simulink model "Timers"  (R2025a)
settings: Solver=FixedStepDiscrete  StartTime=0  StopTime=1  FixedStep=1e-7  RelTol=1e-3
libraries: simulink_extras x216, simulink x13
(part 1 of 7)
settings Model: PacingRate=0.000500  Creator=Erys  LastModifiedBy=Erys
settings DebuggingCC: AlgebraicLoopMsg=none  ForceCombineOutputUpdateInSim=on

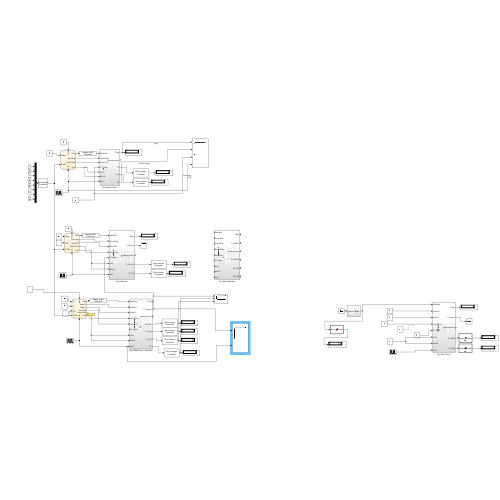
[thumbnail: Simulink's stored preview of the top-level diagram]
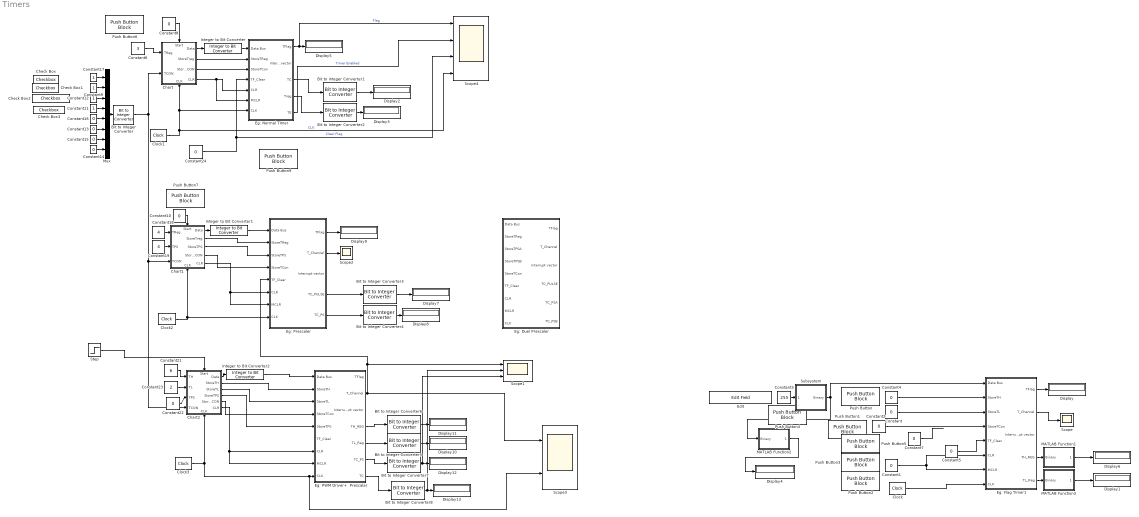
== system Timers ==
  Bit to Integer Converter : simulink/Logic and Bit Operations/Bit to Integer Converter  nbits=8  bitOrder=MSB first  signedOutputValues=Unsigned  outDtype=double  outDtypeSigned=Inherit via internal rule
  Bit to Integer Converter{1..8} (8 alike) : simulink/Logic and Bit Operations/Bit to Integer Converter  nbits=8  bitOrder=MSB first  signedOutputValues=Unsigned  outDtype=Inherit via internal rule  outDtypeSigned=Inherit via internal rule
  Chart : Stateflow chart  TreatAsAtomicUnit=on
      settings: PortSchema="{\"entries\":[{\"content\":{\"sides\":[{\"content\":{\"connectorIds\":[\"In4\",\"In1\"]},\"type\":\"ConnectorPlacement.EquallySpacedRectSide\",\"uuid\":\"e074c012-5276-4155-8d53-51c993f7710d\"},{\"content\":{\"connectorIds\":[\"Out2\",\"Out3\",\"Out4\",\"Out1\"],\"side\":\"RIGHT\"},\"type\":\"ConnectorPlacement.EquallySpacedRectSide\",\"uuid\":\"84a6596f-ad90-40d7-98bc-5213cd18cdfd\"},{\"content\":{\"connectorIds\":[\"In2\"],\"side\":\"TOP\"},\"type\":\"ConnectorPlacement.EquallySpacedRectSide\",\"uuid\":\"9e281591-ea24-4a8d-8cd5-85def40d3d51\"},{\"content\":{\"connectorIds\":[\"In3\"],\"side\":\"BOTTOM\"},\"type\":\"ConnectorPlacement.EquallySpacedRectSide\",\"uuid\":\"88479451-5760-4ccc-a9c9-4ac76de2b8f0\"}]},\"type\":\"ConnectorPlacement.EquallySpacedConnector\",\"uuid\":\"45dca767-207d-4cb9-a557-26c3450393e5\"}],\"packageUris\":[\"http://schema.mathworks.com/mf0/Connector/R2020b\"],\"version\":\"1.0\"}"
  Chart1 : Stateflow chart  TreatAsAtomicUnit=on
      settings: PortSchema="{\"entries\":[{\"content\":{\"sides\":[{\"content\":{\"connectorIds\":[\"In4\",\"In5\",\"In1\"]},\"type\":\"ConnectorPlacement.EquallySpacedRectSide\",\"uuid\":\"e074c012-5276-4155-8d53-51c993f7710d\"},{\"content\":{\"connectorIds\":[\"Out2\",\"Out4\",\"Out3\",\"Out5\",\"Out1\"],\"side\":\"RIGHT\"},\"type\":\"ConnectorPlacement.EquallySpacedRectSide\",\"uuid\":\"84a6596f-ad90-40d7-98bc-5213cd18cdfd\"},{\"content\":{\"connectorIds\":[\"In2\"],\"side\":\"TOP\"},\"type\":\"ConnectorPlacement.EquallySpacedRectSide\",\"uuid\":\"9e281591-ea24-4a8d-8cd5-85def40d3d51\"},{\"content\":{\"connectorIds\":[\"In3\"],\"side\":\"BOTTOM\"},\"type\":\"ConnectorPlacement.EquallySpacedRectSide\",\"uuid\":\"88479451-5760-4ccc-a9c9-4ac76de2b8f0\"}]},\"type\":\"ConnectorPlacement.EquallySpacedConnector\",\"uuid\":\"45dca767-207d-4cb9-a557-26c3450393e5\"}],\"packageUris\":[\"http://schema.mathworks.com/mf0/Connector/R2020b\"],\"version\":\"1.0\"}"
  Chart2 : Stateflow chart  TreatAsAtomicUnit=on
      settings: PortSchema="{\"entries\":[{\"content\":{\"sides\":[{\"content\":{\"connectorIds\":[\"In4\",\"In6\",\"In5\",\"In1\"]},\"type\":\"ConnectorPlacement.EquallySpacedRectSide\",\"uuid\":\"e074c012-5276-4155-8d53-51c993f7710d\"},{\"content\":{\"connectorIds\":[\"Out2\",\"Out5\",\"Out6\",\"Out3\",\"Out4\",\"Out1\"],\"side\":\"RIGHT\"},\"type\":\"ConnectorPlacement.EquallySpacedRectSide\",\"uuid\":\"84a6596f-ad90-40d7-98bc-5213cd18cdfd\"},{\"content\":{\"connectorIds\":[\"In2\"],\"side\":\"TOP\"},\"type\":\"ConnectorPlacement.EquallySpacedRectSide\",\"uuid\":\"9e281591-ea24-4a8d-8cd5-85def40d3d51\"},{\"content\":{\"connectorIds\":[\"In3\"],\"side\":\"BOTTOM\"},\"type\":\"ConnectorPlacement.EquallySpacedRectSide\",\"uuid\":\"88479451-5760-4ccc-a9c9-4ac76de2b8f0\"}]},\"type\":\"ConnectorPlacement.EquallySpacedConnector\",\"uuid\":\"45dca767-207d-4cb9-a557-26c3450393e5\"}],\"packageUris\":[\"http://schema.mathworks.com/mf0/Connector/R2020b\"],\"version\":\"1.0\"}"
  Check Box : Checkbox  LabelPosition=Hide  ShowInitialText=on  Label=Enable  Values=[0.0, 1.0]
  Check Box1 : Checkbox  LabelPosition=Hide  ShowInitialText=on  Label=AutoReload  Values=[0.0, 1.0]
  Check Box2 : Checkbox  LabelPosition=Hide  ShowInitialText=on  Label=INterrupt  Values=[0.0, 1.0]
  Check Box3 : Checkbox  LabelPosition=Hide  ShowInitialText=on  Label=Gate  Values=[0.0, 1.0]
  Clock : simulink_extras/Flip Flops/Clock  period=0.01
  Clock1 : simulink_extras/Flip Flops/Clock  period=0.001
  Clock2 : simulink_extras/Flip Flops/Clock  period=0.0001
  Clock3 : simulink_extras/Flip Flops/Clock  period=0.0001
  Constant{,1..2,4..5,7,13..16} (10 alike) : Constant  Value=0  OutDataTypeStr=boolean
  Constant{8,10,22,24} (4 alike) : Constant  Value=0
  Constant{9,11..12,17} (4 alike) : Constant  OutDataTypeStr=boolean
  Constant18 : Constant  Value=4
  Constant19 : Constant  Value=4
  Constant21 : Constant  Value=6
  Constant23 : Constant  Value=2
  Constant3 : Constant  Value=255
  Constant6 : Constant  Value=3
  Display{,1..13} (14 alike) : Display
  Edit : EditField  LabelPosition=Hide  ShowInitialText=on  Alignment=Center
  Eg: Duel Prescaler : Subsystem
  Eg: Flag Timer1 : Subsystem
  Eg: Normal TImer : Subsystem
  Eg: PWM Driver+  Prescalar : Subsystem
  Eg: Prescaler : Subsystem
  Integer to Bit Converter : simulink/Logic and Bit Operations/Integer to Bit Converter  nbits=8  signedInputValues=Unsigned  bitOrder=MSB first  outDtype=Inherit via internal rule
  Integer to Bit Converter1 : simulink/Logic and Bit Operations/Integer to Bit Converter  nbits=8  signedInputValues=Unsigned  bitOrder=MSB first  outDtype=Inherit via internal rule
  Integer to Bit Converter2 : simulink/Logic and Bit Operations/Integer to Bit Converter  nbits=8  signedInputValues=Unsigned  bitOrder=MSB first  outDtype=Inherit via internal rule
  MATLAB Function1 : MATLAB Function  TreatAsAtomicUnit=on
  MATLAB Function2 : MATLAB Function  TreatAsAtomicUnit=on
  MATLAB Function3 : MATLAB Function  TreatAsAtomicUnit=on
  Mux : Mux  Inputs=8
  Push Button : PushButtonBlock  ButtonText=TH  IconOnColor=[0.0, 0.39215686274509803, 0.0]  IconOffColor=[0.0, 1.0, 0.0]  OffValue=0.000000
  Push Button1 : PushButtonBlock  ButtonText=T_CON  IconOnColor=[0.0, 0.39215686274509803, 0.0]  IconOffColor=[0.0, 1.0, 0.0]  OffValue=0.000000
  Push Button2 : PushButtonBlock  ButtonText=CLR  IconOnColor=[0.0, 0.39215686274509803, 0.0]  IconOffColor=[0.0, 1.0, 0.0]  OffValue=0.000000
  Push Button3 : PushButtonBlock  ButtonText=RST  IconOnColor=[0.0, 0.39215686274509803, 0.0]  IconOffColor=[0.0, 1.0, 0.0]  OffValue=0.000000
  Push Button4 : PushButtonBlock  ButtonText=TL  IconOnColor=[0.0, 0.39215686274509803, 0.0]  IconOffColor=[0.0, 1.0, 0.0]  OffValue=0.000000
  Push Button5 : PushButtonBlock  ButtonText=T_PSB  IconOnColor=[0.0, 0.39215686274509803, 0.0]  IconOffColor=[0.0, 1.0, 0.0]  OffValue=0.000000
  Push Button6 : PushButtonBlock  ButtonText=Start  IconOnColor=[0.0, 0.39215686274509803, 0.0]  IconOffColor=[0.0, 1.0, 0.0]  OffValue=0.000000
  Push Button7 : PushButtonBlock  ButtonText=Start  IconOnColor=[0.0, 0.39215686274509803, 0.0]  IconOffColor=[0.0, 1.0, 0.0]  OffValue=0.000000
  Push Button9 : PushButtonBlock  IconOnColor=[0.0, 0.39215686274509803, 0.0]  IconOffColor=[0.0, 1.0, 0.0]  OffValue=0.000000
  Scope : Scope
      settings: ActiveDisplayYMinimum=-1  ActiveDisplayYMaximum=1
  Scope1 : Scope  NumInputPorts=3
      settings: ActiveDisplayYMinimum=-0.12499999999999997  ActiveDisplayYMaximum=1.125
  Scope2 : Scope
      settings: ActiveDisplayYMinimum=-1  ActiveDisplayYMaximum=1
  Scope3 : Scope  NumInputPorts=2
      settings: ActiveDisplayYMinimum=-0.12499999999999997  ActiveDisplayYMaximum=1.125  DataLoggingVariableName=ScopeData4
  Scope4 : Scope  NumInputPorts=4
      settings: ActiveDisplayString=4  ActiveDisplayYMinimum=-0.12499999999999997  ActiveDisplayYMaximum=1.125  DataLoggingVariableName=ScopeData7
  Step : Step  Time=0.001  SampleTime=0
  Subsystem : Subsystem
  wires:
  Clock/1 -> Eg: Flag Timer1/8(CLK)
  Constant1/1 -> Eg: Flag Timer1/7(MCLR), Eg: Flag Timer1/6(CLR)
  Constant3/1 -> Subsystem/1(Decimal)
  Subsystem/1(Binary) -> MATLAB Function2/1(Binary), Eg: Flag Timer1/1(Data Bus)
  Constant5/1 -> Eg: Flag Timer1/5(TF_Clear)
  MATLAB Function2/1(Decimal) -> Display4/1
  Constant/1 -> Eg: Flag Timer1/3(StoreTL)
  Constant7/1 -> ?
  Constant4/1 -> Eg: Flag Timer1/2(StoreTH)
  Constant2/1 -> Eg: Flag Timer1/4(StoreTCon)
  Eg: Flag Timer1/2(T_Channel) -> Scope/1
  Eg: Flag Timer1/1(TFlag) -> Display/1
  Eg: Flag Timer1/4(TH_REG) -> MATLAB Function1/1(Binary)
  MATLAB Function1/1(Decimal) -> Display6/1
  MATLAB Function3/1(Decimal) -> Display1/1
  Eg: Flag Timer1/5(TL_Reg) -> MATLAB Function3/1(Binary)
  Clock1/1 -> Scope4/4, Chart/3(CLK), Eg: Normal TImer/7(CLK)  "CLK"
  Chart/1(CLR) -> Eg: Normal TImer/5(CLR), Eg: Normal TImer/6(MCLR)
  Constant6/1 -> Chart/4(TReg)
  Constant8/1 -> Chart/2(Start)
  Chart/2(Data) -> Integer to Bit Converter/1
  Integer to Bit Converter/1 -> Eg: Normal TImer/1(Data Bus)
  Chart/3(StoreTreg) -> Eg: Normal TImer/2(StoreTReg)
  Chart/4(StoreTCON) -> Eg: Normal TImer/3(StoreTCon)
  Eg: Normal TImer/3(TC) -> Bit to Integer Converter1/1
  Bit to Integer Converter1/1 -> Display2/1
  Bit to Integer Converter2/1 -> Display3/1
  Eg: Normal TImer/4(Treg) -> Bit to Integer Converter2/1
  Eg: Normal TImer/1(TFlag) -> Scope4/1, Display5/1  "Flag"
  Chart1/2(Data) -> Integer to Bit Converter1/1
  Eg: Prescaler/1(TFlag) -> Display9/1
  Integer to Bit Converter1/1 -> Eg: Prescaler/1(Data Bus)
  Chart1/1(CLR) -> Eg: Prescaler/6(CLR), Eg: Prescaler/7(MCLR)
  Constant10/1 -> Chart1/2(Start)
  Clock2/1 -> Chart1/3(CLK), Eg: Prescaler/8(CLK)
  Eg: Prescaler/2(T_Channel) -> Scope2/1
  Chart1/5(StoreTCON) -> Eg: Prescaler/4(StoreTCon)
  Chart1/4(StoreTreg) -> Eg: Prescaler/2(StoreTReg)
  Chart1/3(StoreTPS) -> Eg: Prescaler/3(StoreTPS)
  Constant16/1 -> Mux/5
  Constant17/1 -> Mux/1
  Constant9/1 -> Mux/2
  Constant12/1 -> Mux/3
  Constant15/1 -> Mux/7
  Constant11/1 -> Mux/4
  Constant14/1 -> Mux/8
  Mux/1 -> Bit to Integer Converter/1
  Constant13/1 -> Mux/6
  Constant18/1 -> Chart1/4(TReg)
  Constant19/1 -> Chart1/5(TPS)
  Bit to Integer Converter3/1 -> Display7/1
  Bit to Integer Converter4/1 -> Display8/1
  Eg: Prescaler/4(TC_PULSE) -> Bit to Integer Converter3/1
  Eg: Prescaler/5(TC_PS) -> Bit to Integer Converter4/1
  Constant22/1 -> Chart2/5(TPS)
  Bit to Integer Converter/1 -> Chart2/1(TCON), Chart1/1(TCON), Chart/1(TCON)
  Clock3/1 -> Scope3/2, Eg: PWM Driver+  Prescalar/9(CLK), Chart2/3(CLK)
  Integer to Bit Converter2/1 -> Eg: PWM Driver+  Prescalar/1(Data Bus)
  Chart2/2(Data) -> Integer to Bit Converter2/1
  Chart2/1(CLR) -> Eg: PWM Driver+  Prescalar/8(MCLR), Eg: PWM Driver+  Prescalar/7(CLR)
  Constant21/1 -> Chart2/4(TH)
  Chart2/5(StoreTH) -> Eg: PWM Driver+  Prescalar/2(StoreTH)
  Chart2/6(StoreTL) -> Eg: PWM Driver+  Prescalar/3(StoreTL)
  Chart2/3(StoreTPS) -> Eg: PWM Driver+  Prescalar/5(StoreTPS)
  Chart2/4(StoreTCON) -> Eg: PWM Driver+  Prescalar/4(StoreTCon)
  Constant23/1 -> Chart2/6(TL)
  Eg: PWM Driver+  Prescalar/2(T_Channel) -> Scope3/1, Eg: Prescaler/5(TF_Clear), Scope1/1
  Eg: PWM Driver+  Prescalar/5(TL_Reg) -> Bit to Integer Converter5/1
  Bit to Integer Converter5/1 -> Display10/1
  Eg: PWM Driver+  Prescalar/4(TH_REG) -> Bit to Integer Converter6/1
  Bit to Integer Converter6/1 -> Display11/1
  Bit to Integer Converter7/1 -> Scope1/3, Display12/1
  Eg: PWM Driver+  Prescalar/6(TC_PS) -> Bit to Integer Converter7/1
  Bit to Integer Converter8/1 -> Scope1/2, Display13/1
  Eg: PWM Driver+  Prescalar/7(TC) -> Bit to Integer Converter8/1
  Step/1 -> Chart2/2(Start)
  Eg: Normal TImer/5(TE) -> Scope4/2  "Timer Enabled"
  Constant24/1 -> Scope4/3, Eg: Normal TImer/4(TF_Clear)  "Clear Flag"

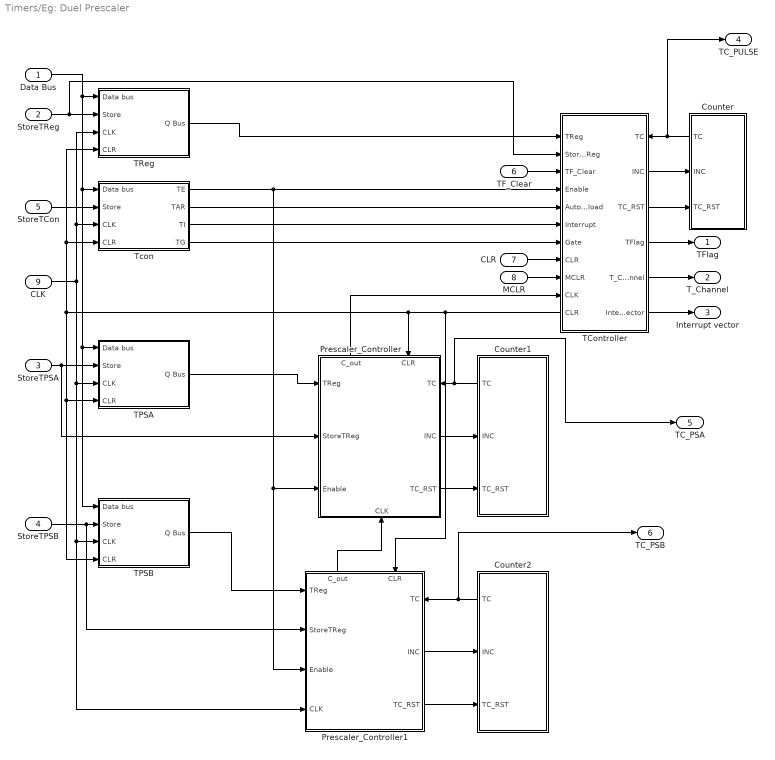
== system Timers/Eg: Duel Prescaler ==
  Data Bus : Inport
  StoreTReg : Inport  Port=2
  StoreTPSA : Inport  Port=3
  StoreTPSB : Inport  Port=4
  StoreTCon : Inport  Port=5
  TF_Clear : Inport  Port=6
  CLR : Inport  Port=7
  MCLR : Inport  Port=8
  CLK : Inport  Port=9
  Counter : Subsystem
      settings: PortSchema="{\"entries\":[{\"content\":{\"sides\":[{\"content\":{\"connectorIds\":[\"Out1\",\"In1\",\"In2\"]},\"type\":\"ConnectorPlacement.EquallySpacedRectSide\",\"uuid\":\"d2ca064e-8e65-4383-9509-923487f0994b\"},{\"content\":{\"side\":\"RIGHT\"},\"type\":\"ConnectorPlacement.EquallySpacedRectSide\",\"uuid\":\"c8a688a5-ee2c-4fad-a889-c5e09b1c269e\"},{\"content\":{\"side\":\"TOP\"},\"type\":\"ConnectorPlacement.EquallySpacedRectSide\",\"uuid\":\"2f0d42e7-9a85-4a58-8ec6-3b7b9eab62de\"},{\"content\":{\"side\":\"BOTTOM\"},\"type\":\"ConnectorPlacement.EquallySpacedRectSide\",\"uuid\":\"38510fd4-2d07-404d-8bb1-895f71011c48\"}]},\"type\":\"ConnectorPlacement.EquallySpacedConnector\",\"uuid\":\"c9cdc40f-5296-4098-a99e-74109d120565\"}],\"packageUris\":[\"http://schema.mathworks.com/mf0/Connector/R2020b\"],\"version\":\"1.0\"}"
  Counter1 : Subsystem
      settings: PortSchema="{\"entries\":[{\"content\":{\"sides\":[{\"content\":{\"connectorIds\":[\"Out1\",\"In1\",\"In2\"]},\"type\":\"ConnectorPlacement.EquallySpacedRectSide\",\"uuid\":\"d2ca064e-8e65-4383-9509-923487f0994b\"},{\"content\":{\"side\":\"RIGHT\"},\"type\":\"ConnectorPlacement.EquallySpacedRectSide\",\"uuid\":\"c8a688a5-ee2c-4fad-a889-c5e09b1c269e\"},{\"content\":{\"side\":\"TOP\"},\"type\":\"ConnectorPlacement.EquallySpacedRectSide\",\"uuid\":\"2f0d42e7-9a85-4a58-8ec6-3b7b9eab62de\"},{\"content\":{\"side\":\"BOTTOM\"},\"type\":\"ConnectorPlacement.EquallySpacedRectSide\",\"uuid\":\"38510fd4-2d07-404d-8bb1-895f71011c48\"}]},\"type\":\"ConnectorPlacement.EquallySpacedConnector\",\"uuid\":\"c9cdc40f-5296-4098-a99e-74109d120565\"}],\"packageUris\":[\"http://schema.mathworks.com/mf0/Connector/R2020b\"],\"version\":\"1.0\"}"
  Counter2 : Subsystem
      settings: PortSchema="{\"entries\":[{\"content\":{\"sides\":[{\"content\":{\"connectorIds\":[\"Out1\",\"In1\",\"In2\"]},\"type\":\"ConnectorPlacement.EquallySpacedRectSide\",\"uuid\":\"d2ca064e-8e65-4383-9509-923487f0994b\"},{\"content\":{\"side\":\"RIGHT\"},\"type\":\"ConnectorPlacement.EquallySpacedRectSide\",\"uuid\":\"c8a688a5-ee2c-4fad-a889-c5e09b1c269e\"},{\"content\":{\"side\":\"TOP\"},\"type\":\"ConnectorPlacement.EquallySpacedRectSide\",\"uuid\":\"2f0d42e7-9a85-4a58-8ec6-3b7b9eab62de\"},{\"content\":{\"side\":\"BOTTOM\"},\"type\":\"ConnectorPlacement.EquallySpacedRectSide\",\"uuid\":\"38510fd4-2d07-404d-8bb1-895f71011c48\"}]},\"type\":\"ConnectorPlacement.EquallySpacedConnector\",\"uuid\":\"c9cdc40f-5296-4098-a99e-74109d120565\"}],\"packageUris\":[\"http://schema.mathworks.com/mf0/Connector/R2020b\"],\"version\":\"1.0\"}"
  Prescaler_Controller : Subsystem
      settings: PortSchema="{\"entries\":[{\"content\":{\"sides\":[{\"content\":{\"connectorIds\":[\"In1\",\"In2\",\"In3\"]},\"type\":\"ConnectorPlacement.EquallySpacedRectSide\",\"uuid\":\"82b85bc6-964b-49ee-8a4b-3356bfec1aee\"},{\"content\":{\"connectorIds\":[\"In6\",\"Out1\",\"Out2\"],\"side\":\"RIGHT\"},\"type\":\"ConnectorPlacement.EquallySpacedRectSide\",\"uuid\":\"8c4af632-7d6e-4ec6-a03e-f6796e56340c\"},{\"content\":{\"connectorIds\":[\"Out3\",\"In4\"],\"side\":\"TOP\"},\"type\":\"ConnectorPlacement.EquallySpacedRectSide\",\"uuid\":\"c668d65a-8355-4e30-8ca9-8213ac4eb35c\"},{\"content\":{\"connectorIds\":[\"In5\"],\"side\":\"BOTTOM\"},\"type\":\"ConnectorPlacement.EquallySpacedRectSide\",\"uuid\":\"7e82bb91-fecf-4aec-a971-3b22643d51d5\"}]},\"type\":\"ConnectorPlacement.EquallySpacedConnector\",\"uuid\":\"0a0bd963-09d6-4454-bda2-144190581a2a\"}],\"packageUris\":[\"http://schema.mathworks.com/mf0/Connector/R2020b\"],\"version\":\"1.0\"}"
  Prescaler_Controller1 : Subsystem
      settings: PortSchema="{\"entries\":[{\"content\":{\"sides\":[{\"content\":{\"connectorIds\":[\"In1\",\"In2\",\"In3\",\"In4\"]},\"type\":\"ConnectorPlacement.EquallySpacedRectSide\",\"uuid\":\"82b85bc6-964b-49ee-8a4b-3356bfec1aee\"},{\"content\":{\"connectorIds\":[\"In6\",\"Out1\",\"Out2\"],\"side\":\"RIGHT\"},\"type\":\"ConnectorPlacement.EquallySpacedRectSide\",\"uuid\":\"8c4af632-7d6e-4ec6-a03e-f6796e56340c\"},{\"content\":{\"connectorIds\":[\"Out3\",\"In5\"],\"side\":\"TOP\"},\"type\":\"ConnectorPlacement.EquallySpacedRectSide\",\"uuid\":\"c668d65a-8355-4e30-8ca9-8213ac4eb35c\"},{\"content\":{\"side\":\"BOTTOM\"},\"type\":\"ConnectorPlacement.EquallySpacedRectSide\",\"uuid\":\"7e82bb91-fecf-4aec-a971-3b22643d51d5\"}]},\"type\":\"ConnectorPlacement.EquallySpacedConnector\",\"uuid\":\"0a0bd963-09d6-4454-bda2-144190581a2a\"}],\"packageUris\":[\"http://schema.mathworks.com/mf0/Connector/R2020b\"],\"version\":\"1.0\"}"
  TController : Subsystem
      settings: PortSchema="{\"entries\":[{\"content\":{\"sides\":[{\"content\":{\"connectorIds\":[\"In1\",\"In2\",\"In3\",\"In4\",\"In5\",\"In6\",\"In7\",\"In8\",\"In9\",\"In10\",\"Out6\"]},\"type\":\"ConnectorPlacement.EquallySpacedRectSide\",\"uuid\":\"82b85bc6-964b-49ee-8a4b-3356bfec1aee\"},{\"content\":{\"connectorIds\":[\"In11\",\"Out1\",\"Out2\",\"Out3\",\"Out4\",\"Out5\"],\"side\":\"RIGHT\"},\"type\":\"ConnectorPlacement.EquallySpacedRectSide\",\"uuid\":\"8c4af632-7d6e-4ec6-a03e-f6796e56340c\"},{\"content\":{\"side\":\"TOP\"},\"type\":\"ConnectorPlacement.EquallySpacedRectSide\",\"uuid\":\"c668d65a-8355-4e30-8ca9-8213ac4eb35c\"},{\"content\":{\"side\":\"BOTTOM\"},\"type\":\"ConnectorPlacement.EquallySpacedRectSide\",\"uuid\":\"7e82bb91-fecf-4aec-a971-3b22643d51d5\"}]},\"type\":\"ConnectorPlacement.EquallySpacedConnector\",\"uuid\":\"0a0bd963-09d6-4454-bda2-144190581a2a\"}],\"packageUris\":[\"http://schema.mathworks.com/mf0/Connector/R2020b\"],\"version\":\"1.0\"}"
  TPSA : Subsystem
  TPSB : Subsystem
  TReg : Subsystem
  Tcon : Subsystem
  TFlag : Outport
  T_Channel : Outport  Port=2
  Interrupt vector : Outport  Port=3
  TC_PULSE : Outport  Port=4
  TC_PSA : Outport  Port=5
  TC_PSB : Outport  Port=6
  wires:
  StoreTReg/1 -> TController/2(StoreTReg), TReg/2(Store)
  Data Bus/1 -> TPSB/1(Data bus), TPSA/1(Data bus), Tcon/1(Data bus), TReg/1(Data bus)
  CLK/1 -> Prescaler_Controller1/4(CLK), TPSB/3(CLK), TPSA/3(CLK), TReg/3(CLK), Tcon/3(CLK)
  TReg/1("Q Bus ") -> TController/1(TReg)
  TController/3(TFlag) -> TFlag/1
  Counter/1(TC) -> TC_PULSE/1, TController/11(TC)
  TController/1(INC) -> Counter/1(INC)
  TF_Clear/1 -> TController/3(TF_Clear)
  StoreTCon/1 -> Tcon/2(Store)
  Tcon/1(TE) -> Prescaler_Controller1/3(Enable), Prescaler_Controller/3(Enable), TController/4(Enable)
  CLR/1 -> TController/8("CLR ")
  MCLR/1 -> TController/9(MCLR)
  Tcon/3(TI) -> TController/6(Interrupt)
  Tcon/4(TG) -> TController/7(Gate)
  TController/5(Interrupt vector) -> Interrupt vector/1
  TController/4(T_Channel) -> T_Channel/1
  TController/6(CLR) -> TReg/4(CLR), Tcon/4(CLR), TPSB/4(CLR), TPSA/4(CLR), Prescaler_Controller/4("CLR "), Prescaler_Controller1/5("CLR ")
  Tcon/2(TAR) -> TController/5(Auto reload)
  TController/2(TC_RST) -> Counter/2(TC_RST)
  StoreTPSA/1 -> Prescaler_Controller/2(StoreTReg), TPSA/2(Store)
  TPSA/1("Q Bus ") -> Prescaler_Controller/1(TReg)
  Prescaler_Controller/1(INC) -> Counter1/1(INC)
  Prescaler_Controller/2(TC_RST) -> Counter1/2(TC_RST)
  Prescaler_Controller/3(C_out) -> TController/10(CLK)
  Counter1/1(TC) -> TC_PSA/1, Prescaler_Controller/6(TC)
  StoreTPSB/1 -> Prescaler_Controller1/2(StoreTReg), TPSB/2(Store)
  Prescaler_Controller1/2(TC_RST) -> Counter2/2(TC_RST)
  Prescaler_Controller1/1(INC) -> Counter2/1(INC)
  TPSB/1("Q Bus ") -> Prescaler_Controller1/1(TReg)
  Prescaler_Controller1/3(C_out) -> Prescaler_Controller/5(CLK)
  Counter2/1(TC) -> Prescaler_Controller1/6(TC), TC_PSB/1

== system Timers/Eg: Flag Timer1 ==
  Data Bus : Inport
  StoreTH : Inport  Port=2
  StoreTL : Inport  Port=3
  StoreTCon : Inport  Port=4
  TF_Clear : Inport  Port=5
  CLR : Inport  Port=6
  MCLR : Inport  Port=7
  CLK : Inport  Port=8
  Counter : Subsystem
      settings: PortSchema="{\"entries\":[{\"content\":{\"sides\":[{\"content\":{\"connectorIds\":[\"Out1\",\"In1\",\"In2\"]},\"type\":\"ConnectorPlacement.EquallySpacedRectSide\",\"uuid\":\"d2ca064e-8e65-4383-9509-923487f0994b\"},{\"content\":{\"side\":\"RIGHT\"},\"type\":\"ConnectorPlacement.EquallySpacedRectSide\",\"uuid\":\"c8a688a5-ee2c-4fad-a889-c5e09b1c269e\"},{\"content\":{\"side\":\"TOP\"},\"type\":\"ConnectorPlacement.EquallySpacedRectSide\",\"uuid\":\"2f0d42e7-9a85-4a58-8ec6-3b7b9eab62de\"},{\"content\":{\"side\":\"BOTTOM\"},\"type\":\"ConnectorPlacement.EquallySpacedRectSide\",\"uuid\":\"38510fd4-2d07-404d-8bb1-895f71011c48\"}]},\"type\":\"ConnectorPlacement.EquallySpacedConnector\",\"uuid\":\"c9cdc40f-5296-4098-a99e-74109d120565\"}],\"packageUris\":[\"http://schema.mathworks.com/mf0/Connector/R2020b\"],\"version\":\"1.0\"}"
  TController : Subsystem
      settings: PortSchema="{\"entries\":[{\"content\":{\"sides\":[{\"content\":{\"connectorIds\":[\"In1\",\"In2\",\"In3\",\"In4\",\"In5\",\"In6\",\"In7\",\"In8\",\"In9\",\"In10\",\"In11\",\"In12\",\"Out6\"]},\"type\":\"ConnectorPlacement.EquallySpacedRectSide\",\"uuid\":\"82b85bc6-964b-49ee-8a4b-3356bfec1aee\"},{\"content\":{\"connectorIds\":[\"In13\",\"Out1\",\"Out2\",\"Out3\",\"Out4\",\"Out5\"],\"side\":\"RIGHT\"},\"type\":\"ConnectorPlacement.EquallySpacedRectSide\",\"uuid\":\"8c4af632-7d6e-4ec6-a03e-f6796e56340c\"},{\"content\":{\"side\":\"TOP\"},\"type\":\"ConnectorPlacement.EquallySpacedRectSide\",\"uuid\":\"c668d65a-8355-4e30-8ca9-8213ac4eb35c\"},{\"content\":{\"side\":\"BOTTOM\"},\"type\":\"ConnectorPlacement.EquallySpacedRectSide\",\"uuid\":\"7e82bb91-fecf-4aec-a971-3b22643d51d5\"}]},\"type\":\"ConnectorPlacement.EquallySpacedConnector\",\"uuid\":\"0a0bd963-09d6-4454-bda2-144190581a2a\"}],\"packageUris\":[\"http://schema.mathworks.com/mf0/Connector/R2020b\"],\"version\":\"1.0\"}"
  TH : Subsystem
  TL : Subsystem
  Tcon : Subsystem
  TFlag : Outport
  T_Channel : Outport  Port=2
  Interrupt vector : Outport  Port=3
  TH_REG : Outport  Port=4
  TL_Reg : Outport  Port=5
  wires:
  StoreTL/1 -> TController/3(StoreTL), TL/2(Store)
  Data Bus/1 -> Tcon/1(Data bus), TL/1(Data bus), TH/1(Data bus)
  CLK/1 -> TL/3(CLK), TH/3(CLK), Tcon/3(CLK), TController/12(CLK)
  TL/1("Q Bus ") -> TController/4(TL_Reg), TL_Reg/1
  TController/3(TFlag) -> TFlag/1
  Counter/1(TC) -> TController/13(TC)
  TController/1(INC) -> Counter/1(INC)
  TF_Clear/1 -> TController/5(TF_Clear)
  StoreTCon/1 -> Tcon/2(Store)
  Tcon/1(TE) -> TController/6(Enable)
  CLR/1 -> TController/10("CLR ")
  MCLR/1 -> TController/11(MCLR)
  Tcon/3(TI) -> TController/8(Interrupt)
  Tcon/4(TG) -> TController/9(Gate)
  TController/5(Interrupt vector) -> Interrupt vector/1
  TController/4(T_Channel) -> T_Channel/1
  TController/6(CLR) -> TH/4(CLR), TL/4(CLR), Tcon/4(CLR)
  Tcon/2(TAR) -> TController/7(Auto reload)
  TController/2(TC_RST) -> Counter/2(TC_RST)
  StoreTH/1 -> TController/2(StoreTH), TH/2(Store)
  TH/1("Q Bus ") -> TH_REG/1, TController/1(TH_Reg)

== system Timers/Eg: Normal TImer ==
  Data Bus : Inport
  StoreTReg : Inport  Port=2
  StoreTCon : Inport  Port=3
  TF_Clear : Inport  Port=4
  CLR : Inport  Port=5
  MCLR : Inport  Port=6
  CLK : Inport  Port=7
  Bit to Integer Converter1 : simulink/Logic and Bit Operations/Bit to Integer Converter  nbits=8  bitOrder=MSB first  signedOutputValues=Unsigned  outDtype=Inherit via internal rule  outDtypeSigned=Inherit via internal rule
  Counter : Subsystem
      settings: PortSchema="{\"entries\":[{\"content\":{\"sides\":[{\"content\":{\"connectorIds\":[\"Out1\",\"In1\",\"In2\"]},\"type\":\"ConnectorPlacement.EquallySpacedRectSide\",\"uuid\":\"d2ca064e-8e65-4383-9509-923487f0994b\"},{\"content\":{\"side\":\"RIGHT\"},\"type\":\"ConnectorPlacement.EquallySpacedRectSide\",\"uuid\":\"c8a688a5-ee2c-4fad-a889-c5e09b1c269e\"},{\"content\":{\"side\":\"TOP\"},\"type\":\"ConnectorPlacement.EquallySpacedRectSide\",\"uuid\":\"2f0d42e7-9a85-4a58-8ec6-3b7b9eab62de\"},{\"content\":{\"side\":\"BOTTOM\"},\"type\":\"ConnectorPlacement.EquallySpacedRectSide\",\"uuid\":\"38510fd4-2d07-404d-8bb1-895f71011c48\"}]},\"type\":\"ConnectorPlacement.EquallySpacedConnector\",\"uuid\":\"c9cdc40f-5296-4098-a99e-74109d120565\"}],\"packageUris\":[\"http://schema.mathworks.com/mf0/Connector/R2020b\"],\"version\":\"1.0\"}"
  Delay One Step : Delay  DelayLength=1  SampleTime=1e-6
  Display2 : Display
  TController : Subsystem
      settings: PortSchema="{\"entries\":[{\"content\":{\"sides\":[{\"content\":{\"connectorIds\":[\"In1\",\"In2\",\"In3\",\"In4\",\"In5\",\"In6\",\"In7\",\"In8\",\"Out5\"]},\"type\":\"ConnectorPlacement.EquallySpacedRectSide\",\"uuid\":\"82b85bc6-964b-49ee-8a4b-3356bfec1aee\"},{\"content\":{\"connectorIds\":[\"In10\",\"Out1\",\"Out2\",\"Out3\",\"Out4\"],\"side\":\"RIGHT\"},\"type\":\"ConnectorPlacement.EquallySpacedRectSide\",\"uuid\":\"8c4af632-7d6e-4ec6-a03e-f6796e56340c\"},{\"content\":{\"side\":\"TOP\"},\"type\":\"ConnectorPlacement.EquallySpacedRectSide\",\"uuid\":\"c668d65a-8355-4e30-8ca9-8213ac4eb35c\"},{\"content\":{\"connectorIds\":[\"In9\"],\"side\":\"BOTTOM\"},\"type\":\"ConnectorPlacement.EquallySpacedRectSide\",\"uuid\":\"7e82bb91-fecf-4aec-a971-3b22643d51d5\"}]},\"type\":\"ConnectorPlacement.EquallySpacedConnector\",\"uuid\":\"0a0bd963-09d6-4454-bda2-144190581a2a\"}],\"packageUris\":[\"http://schema.mathworks.com/mf0/Connector/R2020b\"],\"version\":\"1.0\"}"
  TReg : Subsystem
  Tcon : Subsystem
  TFlag : Outport
  Interrupt vector : Outport  Port=2
  TC : Outport  Port=3
  Treg : Outport  Port=4
  TE : Outport  Port=5
  wires:
  StoreTReg/1 -> TReg/2(Store)
  Data Bus/1 -> TReg/1(Data bus), Tcon/1(Data bus)
  CLK/1 -> TController/9(MainCLK), TController/8(CLK_IN), TReg/3(CLK), Tcon/3(CLK)
  TReg/1("Q Bus ") -> TController/1(TReg), Treg/1
  TController/3(TFlag) -> TFlag/1
  Counter/1(TC) -> Bit to Integer Converter1/1, Delay One Step/1
  TController/1(INC) -> Counter/1(INC)
  TF_Clear/1 -> TController/3(TF_Clear)
  StoreTCon/1 -> TController/2(StoreTCON), Tcon/2(Store)
  Tcon/1(TE) -> TE/1, TController/4(Enable)
  CLR/1 -> TController/6("CLR ")
  MCLR/1 -> TController/7(MCLR)
  Tcon/3(TI) -> TController/5(Interrupt)
  TController/4(Interrupt vector) -> Interrupt vector/1
  TController/5(TMR_CLR) -> TReg/4(CLR), Tcon/4(CLR)
  TController/2(TC_RST) -> Counter/2(TC_RST)
  Delay One Step/1 -> TC/1, TController/10(TC)
  Bit to Integer Converter1/1 -> Display2/1

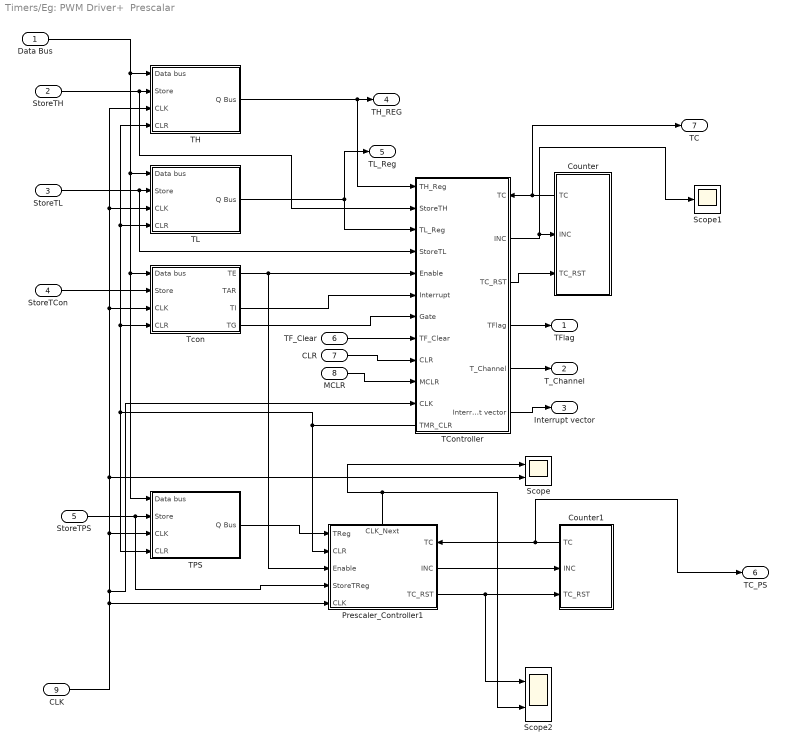
== system Timers/Eg: PWM Driver+  Prescalar ==
  Data Bus : Inport
  StoreTH : Inport  Port=2
  StoreTL : Inport  Port=3
  StoreTCon : Inport  Port=4
  StoreTPS : Inport  Port=5
  TF_Clear : Inport  Port=6
  CLR : Inport  Port=7
  MCLR : Inport  Port=8
  CLK : Inport  Port=9
  Counter : Subsystem
      settings: PortSchema="{\"entries\":[{\"content\":{\"sides\":[{\"content\":{\"connectorIds\":[\"Out1\",\"In1\",\"In2\"]},\"type\":\"ConnectorPlacement.EquallySpacedRectSide\",\"uuid\":\"d2ca064e-8e65-4383-9509-923487f0994b\"},{\"content\":{\"side\":\"RIGHT\"},\"type\":\"ConnectorPlacement.EquallySpacedRectSide\",\"uuid\":\"c8a688a5-ee2c-4fad-a889-c5e09b1c269e\"},{\"content\":{\"side\":\"TOP\"},\"type\":\"ConnectorPlacement.EquallySpacedRectSide\",\"uuid\":\"2f0d42e7-9a85-4a58-8ec6-3b7b9eab62de\"},{\"content\":{\"side\":\"BOTTOM\"},\"type\":\"ConnectorPlacement.EquallySpacedRectSide\",\"uuid\":\"38510fd4-2d07-404d-8bb1-895f71011c48\"}]},\"type\":\"ConnectorPlacement.EquallySpacedConnector\",\"uuid\":\"c9cdc40f-5296-4098-a99e-74109d120565\"}],\"packageUris\":[\"http://schema.mathworks.com/mf0/Connector/R2020b\"],\"version\":\"1.0\"}"
  Counter1 : Subsystem
      settings: PortSchema="{\"entries\":[{\"content\":{\"sides\":[{\"content\":{\"connectorIds\":[\"Out1\",\"In1\",\"In2\"]},\"type\":\"ConnectorPlacement.EquallySpacedRectSide\",\"uuid\":\"d2ca064e-8e65-4383-9509-923487f0994b\"},{\"content\":{\"side\":\"RIGHT\"},\"type\":\"ConnectorPlacement.EquallySpacedRectSide\",\"uuid\":\"c8a688a5-ee2c-4fad-a889-c5e09b1c269e\"},{\"content\":{\"side\":\"TOP\"},\"type\":\"ConnectorPlacement.EquallySpacedRectSide\",\"uuid\":\"2f0d42e7-9a85-4a58-8ec6-3b7b9eab62de\"},{\"content\":{\"side\":\"BOTTOM\"},\"type\":\"ConnectorPlacement.EquallySpacedRectSide\",\"uuid\":\"38510fd4-2d07-404d-8bb1-895f71011c48\"}]},\"type\":\"ConnectorPlacement.EquallySpacedConnector\",\"uuid\":\"c9cdc40f-5296-4098-a99e-74109d120565\"}],\"packageUris\":[\"http://schema.mathworks.com/mf0/Connector/R2020b\"],\"version\":\"1.0\"}"
  Prescaler_Controller1 : Subsystem
      settings: PortSchema="{\"entries\":[{\"content\":{\"sides\":[{\"content\":{\"connectorIds\":[\"In1\",\"In2\",\"In3\",\"In4\",\"In5\"]},\"type\":\"ConnectorPlacement.EquallySpacedRectSide\",\"uuid\":\"82b85bc6-964b-49ee-8a4b-3356bfec1aee\"},{\"content\":{\"connectorIds\":[\"In6\",\"Out1\",\"Out2\"],\"side\":\"RIGHT\"},\"type\":\"ConnectorPlacement.EquallySpacedRectSide\",\"uuid\":\"8c4af632-7d6e-4ec6-a03e-f6796e56340c\"},{\"content\":{\"connectorIds\":[\"Out3\"],\"side\":\"TOP\"},\"type\":\"ConnectorPlacement.EquallySpacedRectSide\",\"uuid\":\"c668d65a-8355-4e30-8ca9-8213ac4eb35c\"},{\"content\":{\"side\":\"BOTTOM\"},\"type\":\"ConnectorPlacement.EquallySpacedRectSide\",\"uuid\":\"7e82bb91-fecf-4aec-a971-3b22643d51d5\"}]},\"type\":\"ConnectorPlacement.EquallySpacedConnector\",\"uuid\":\"0a0bd963-09d6-4454-bda2-144190581a2a\"}],\"packageUris\":[\"http://schema.mathworks.com/mf0/Connector/R2020b\"],\"version\":\"1.0\"}"
  Scope : Scope  NumInputPorts=2
      settings: ActiveDisplayYMinimum=-0.12499999999999997  ActiveDisplayYMaximum=1.125  DataLoggingVariableName=ScopeData2
  Scope1 : Scope
      settings: ActiveDisplayYMinimum=-0.125  ActiveDisplayYMaximum=1.125  DataLoggingVariableName=ScopeData3
  Scope2 : Scope  NumInputPorts=2
      settings: ActiveDisplayYMinimum=-1  ActiveDisplayYMaximum=1  DataLoggingVariableName=ScopeData6
  TController : Subsystem
      settings: PortSchema="{\"entries\":[{\"content\":{\"sides\":[{\"content\":{\"connectorIds\":[\"In1\",\"In2\",\"In3\",\"In4\",\"In5\",\"In6\",\"In7\",\"In8\",\"In9\",\"In10\",\"In11\",\"Out6\"]},\"type\":\"ConnectorPlacement.EquallySpacedRectSide\",\"uuid\":\"82b85bc6-964b-49ee-8a4b-3356bfec1aee\"},{\"content\":{\"connectorIds\":[\"In12\",\"Out1\",\"Out2\",\"Out3\",\"Out4\",\"Out5\"],\"side\":\"RIGHT\"},\"type\":\"ConnectorPlacement.EquallySpacedRectSide\",\"uuid\":\"8c4af632-7d6e-4ec6-a03e-f6796e56340c\"},{\"content\":{\"side\":\"TOP\"},\"type\":\"ConnectorPlacement.EquallySpacedRectSide\",\"uuid\":\"c668d65a-8355-4e30-8ca9-8213ac4eb35c\"},{\"content\":{\"side\":\"BOTTOM\"},\"type\":\"ConnectorPlacement.EquallySpacedRectSide\",\"uuid\":\"7e82bb91-fecf-4aec-a971-3b22643d51d5\"}]},\"type\":\"ConnectorPlacement.EquallySpacedConnector\",\"uuid\":\"0a0bd963-09d6-4454-bda2-144190581a2a\"}],\"packageUris\":[\"http://schema.mathworks.com/mf0/Connector/R2020b\"],\"version\":\"1.0\"}"
  TH : Subsystem
  TL : Subsystem
  TPS : Subsystem
  Tcon : Subsystem
  TFlag : Outport
  T_Channel : Outport  Port=2
  Interrupt vector : Outport  Port=3
  TH_REG : Outport  Port=4
  TL_Reg : Outport  Port=5
  TC_PS : Outport  Port=6
  TC : Outport  Port=7
  wires:
  StoreTL/1 -> TController/4(StoreTL), TL/2(Store)
  TL/1("Q Bus ") -> TController/3(TL_Reg), TL_Reg/1
  TController/3(TFlag) -> TFlag/1
  Counter/1(TC) -> TC/1, TController/12(TC)
  TController/1(INC) -> Scope1/1, Counter/1(INC)
  TF_Clear/1 -> TController/8(TF_Clear)
  StoreTCon/1 -> Tcon/2(Store)
  CLR/1 -> TController/9("CLR ")
  MCLR/1 -> TController/10(MCLR)
  Tcon/3(TI) -> TController/6(Interrupt)
  Tcon/4(TG) -> TController/7(Gate)
  TController/5(Interrupt vector) -> Interrupt vector/1
  TController/4(T_Channel) -> T_Channel/1
  TController/2(TC_RST) -> Counter/2(TC_RST)
  StoreTH/1 -> TController/2(StoreTH), TH/2(Store)
  TH/1("Q Bus ") -> TH_REG/1, TController/1(TH_Reg)
  Data Bus/1 -> TPS/1(Data bus), Tcon/1(Data bus), TL/1(Data bus), TH/1(Data bus)
  TController/6(TMR_CLR) -> TH/4(CLR), TL/4(CLR), Tcon/4(CLR), TPS/4(CLR), Prescaler_Controller1/2("CLR ")
  Prescaler_Controller1/1(INC) -> Counter1/1(INC)
  Prescaler_Controller1/2(TC_RST) -> Scope2/1, Counter1/2(TC_RST)
  StoreTPS/1 -> Prescaler_Controller1/4(StoreTReg), TPS/2(Store)
  TPS/1("Q Bus ") -> Prescaler_Controller1/1(TReg)
  Counter1/1(TC) -> Prescaler_Controller1/6(TC), TC_PS/1
  Tcon/1(TE) -> Prescaler_Controller1/3(Enable), TController/5(Enable)
  Prescaler_Controller1/3(CLK_Next) -> Scope2/2, Scope/1
  CLK/1 -> Prescaler_Controller1/5(CLK), TController/11(CLK), Scope/2, TL/3(CLK), TH/3(CLK), Tcon/3(CLK), TPS/3(CLK)

== system Timers/Eg: Prescaler ==
  Data Bus : Inport
  StoreTReg : Inport  Port=2
  StoreTPS : Inport  Port=3
  StoreTCon : Inport  Port=4
  TF_Clear : Inport  Port=5
  CLR : Inport  Port=6
  MCLR : Inport  Port=7
  CLK : Inport  Port=8
  Counter : Subsystem
      settings: PortSchema="{\"entries\":[{\"content\":{\"sides\":[{\"content\":{\"connectorIds\":[\"Out1\",\"In1\",\"In2\"]},\"type\":\"ConnectorPlacement.EquallySpacedRectSide\",\"uuid\":\"d2ca064e-8e65-4383-9509-923487f0994b\"},{\"content\":{\"side\":\"RIGHT\"},\"type\":\"ConnectorPlacement.EquallySpacedRectSide\",\"uuid\":\"c8a688a5-ee2c-4fad-a889-c5e09b1c269e\"},{\"content\":{\"side\":\"TOP\"},\"type\":\"ConnectorPlacement.EquallySpacedRectSide\",\"uuid\":\"2f0d42e7-9a85-4a58-8ec6-3b7b9eab62de\"},{\"content\":{\"side\":\"BOTTOM\"},\"type\":\"ConnectorPlacement.EquallySpacedRectSide\",\"uuid\":\"38510fd4-2d07-404d-8bb1-895f71011c48\"}]},\"type\":\"ConnectorPlacement.EquallySpacedConnector\",\"uuid\":\"c9cdc40f-5296-4098-a99e-74109d120565\"}],\"packageUris\":[\"http://schema.mathworks.com/mf0/Connector/R2020b\"],\"version\":\"1.0\"}"
  Counter1 : Subsystem
      settings: PortSchema="{\"entries\":[{\"content\":{\"sides\":[{\"content\":{\"connectorIds\":[\"Out1\",\"In1\",\"In2\"]},\"type\":\"ConnectorPlacement.EquallySpacedRectSide\",\"uuid\":\"d2ca064e-8e65-4383-9509-923487f0994b\"},{\"content\":{\"side\":\"RIGHT\"},\"type\":\"ConnectorPlacement.EquallySpacedRectSide\",\"uuid\":\"c8a688a5-ee2c-4fad-a889-c5e09b1c269e\"},{\"content\":{\"side\":\"TOP\"},\"type\":\"ConnectorPlacement.EquallySpacedRectSide\",\"uuid\":\"2f0d42e7-9a85-4a58-8ec6-3b7b9eab62de\"},{\"content\":{\"side\":\"BOTTOM\"},\"type\":\"ConnectorPlacement.EquallySpacedRectSide\",\"uuid\":\"38510fd4-2d07-404d-8bb1-895f71011c48\"}]},\"type\":\"ConnectorPlacement.EquallySpacedConnector\",\"uuid\":\"c9cdc40f-5296-4098-a99e-74109d120565\"}],\"packageUris\":[\"http://schema.mathworks.com/mf0/Connector/R2020b\"],\"version\":\"1.0\"}"
  Prescaler_Controller1 : Subsystem
      settings: PortSchema="{\"entries\":[{\"content\":{\"sides\":[{\"content\":{\"connectorIds\":[\"In1\",\"In2\",\"In3\",\"In4\"]},\"type\":\"ConnectorPlacement.EquallySpacedRectSide\",\"uuid\":\"d8b67538-102e-44d7-9e8b-b92b81bf702e\"},{\"content\":{\"connectorIds\":[\"In6\",\"Out1\",\"Out2\"],\"side\":\"RIGHT\"},\"type\":\"ConnectorPlacement.EquallySpacedRectSide\",\"uuid\":\"b22991f5-bd5f-436f-b918-d814cc2c602d\"},{\"content\":{\"connectorIds\":[\"Out3\",\"In5\"],\"side\":\"TOP\"},\"type\":\"ConnectorPlacement.EquallySpacedRectSide\",\"uuid\":\"560bdb7a-9d2d-4e0f-9ca8-ca4e9ca93f58\"}]},\"type\":\"ConnectorPlacement.EquallySpacedConnector\",\"uuid\":\"7dded13d-1636-4ebe-9266-648b23ea5229\"}],\"packageUris\":[\"http://schema.mathworks.com/mf0/Connector/R2020b\"],\"version\":\"1.0\"}"
  Scope : Scope  NumInputPorts=2
      settings: ActiveDisplayYMinimum=-0.12499999999999997  ActiveDisplayYMaximum=1.125  DataLoggingVariableName=ScopeData8
  TController : Subsystem
      settings: PortSchema="{\"entries\":[{\"content\":{\"sides\":[{\"content\":{\"connectorIds\":[\"In1\",\"In2\",\"In3\",\"In4\",\"In5\",\"In6\",\"In7\",\"In8\",\"In9\",\"In10\",\"Out6\"]},\"type\":\"ConnectorPlacement.EquallySpacedRectSide\",\"uuid\":\"82b85bc6-964b-49ee-8a4b-3356bfec1aee\"},{\"content\":{\"connectorIds\":[\"In11\",\"Out1\",\"Out2\",\"Out3\",\"Out4\",\"Out5\"],\"side\":\"RIGHT\"},\"type\":\"ConnectorPlacement.EquallySpacedRectSide\",\"uuid\":\"8c4af632-7d6e-4ec6-a03e-f6796e56340c\"},{\"content\":{\"side\":\"TOP\"},\"type\":\"ConnectorPlacement.EquallySpacedRectSide\",\"uuid\":\"c668d65a-8355-4e30-8ca9-8213ac4eb35c\"},{\"content\":{\"side\":\"BOTTOM\"},\"type\":\"ConnectorPlacement.EquallySpacedRectSide\",\"uuid\":\"7e82bb91-fecf-4aec-a971-3b22643d51d5\"}]},\"type\":\"ConnectorPlacement.EquallySpacedConnector\",\"uuid\":\"0a0bd963-09d6-4454-bda2-144190581a2a\"}],\"packageUris\":[\"http://schema.mathworks.com/mf0/Connector/R2020b\"],\"version\":\"1.0\"}"
  TPS : Subsystem
  TReg : Subsystem
  Tcon : Subsystem
  TFlag : Outport
  T_Channel : Outport  Port=2
  Interrupt vector : Outport  Port=3
  TC_PULSE : Outport  Port=4
  TC_PS : Outport  Port=5
  wires:
  StoreTReg/1 -> TController/1(StoreTReg), TReg/2(Store)
  Data Bus/1 -> TPS/1(Data bus), Tcon/1(Data bus), TReg/1(Data bus)
  CLK/1 -> Scope/2, Prescaler_Controller1/4(CLK), TPS/3(CLK), TReg/3(CLK), Tcon/3(CLK)
  TReg/1("Q Bus ") -> TController/2(TReg)
  TController/3(TFlag) -> TFlag/1
  Counter/1(TC) -> TC_PULSE/1, TController/11(TC)
  TController/1(INC) -> Counter/1(INC)
  TF_Clear/1 -> TController/3(TF_Clear)
  StoreTCon/1 -> Tcon/2(Store)
  Tcon/1(TE) -> Prescaler_Controller1/2(Enable), TController/4(Enable)
  CLR/1 -> TController/8("CLR ")
  MCLR/1 -> TController/9(MCLR)
  Tcon/3(TI) -> TController/6(Interrupt)
  Tcon/4(TG) -> TController/7(Output)
  TController/5(Interrupt vector) -> Interrupt vector/1
  TController/4(T_Channel) -> T_Channel/1
  TController/6(CLR) -> Prescaler_Controller1/5("CLR "), TReg/4(CLR), Tcon/4(CLR), TPS/4(CLR)
  Tcon/2(TAR) -> TController/5(Auto reload)
  TController/2(TC_RST) -> Counter/2(TC_RST)
  StoreTPS/1 -> Prescaler_Controller1/3(StoreTReg), TPS/2(Store)
  TPS/1("Q Bus ") -> Prescaler_Controller1/1(TReg)
  Prescaler_Controller1/1(INC) -> Counter1/1(INC)
  Prescaler_Controller1/2(TC_RST) -> Counter1/2(TC_RST)
  Prescaler_Controller1/3(CLK_Next) -> Scope/1, TController/10(CLK)
  Counter1/1(TC) -> Prescaler_Controller1/6(TC), TC_PS/1

== system Timers/Subsystem ==
  Decimal : Inport
  MATLAB Function : MATLAB Function  TreatAsAtomicUnit=on
  Mux : Mux  Inputs=8
  Binary : Outport
  wires:
  MATLAB Function/5(e) -> Mux/5
  MATLAB Function/7(g) -> Mux/7
  MATLAB Function/1(a) -> Mux/1
  MATLAB Function/2(b) -> Mux/2
  MATLAB Function/4(d) -> Mux/4
  MATLAB Function/8(h) -> Mux/8
  Mux/1 -> Binary/1
  MATLAB Function/3(c) -> Mux/3
  MATLAB Function/6(f) -> Mux/6
  Decimal/1 -> MATLAB Function/1(number)

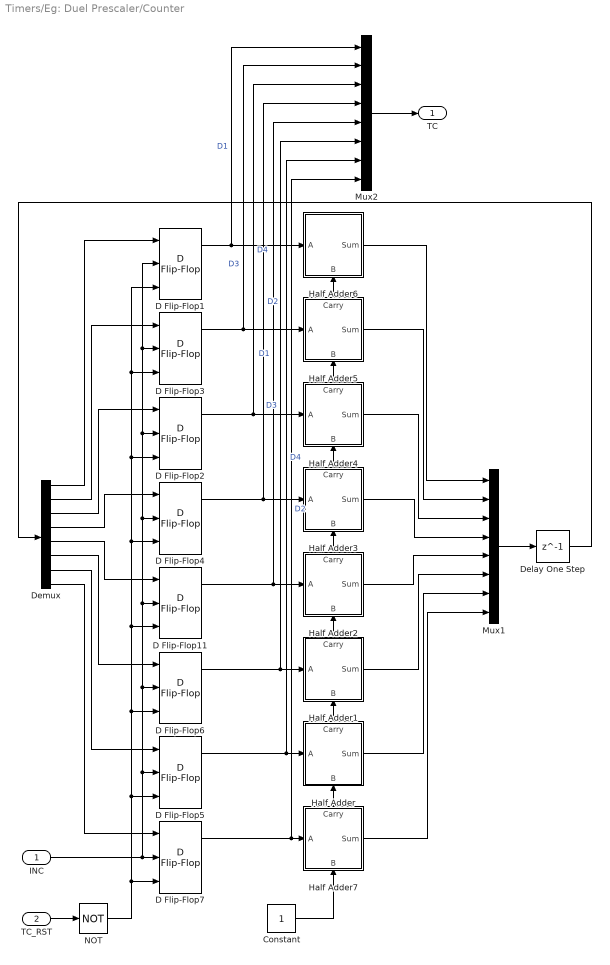
== system Timers/Eg: Duel Prescaler/Counter ==
  INC : Inport
  TC_RST : Inport  Port=2
  Constant : Constant
  D Flip-Flop{1..7,11} (8 alike) : simulink_extras/Flip Flops/D Flip-Flop
  Delay One Step : Delay  DelayLength=1
  Demux : Demux  Outputs=8
  Half Adder : Subsystem
      settings: PortSchema="{\"entries\":[{\"content\":{\"sides\":[{\"content\":{\"connectorIds\":[\"In1\"]},\"type\":\"ConnectorPlacement.EquallySpacedRectSide\",\"uuid\":\"d3a7e232-15f2-47a9-a065-9480c81dc57e\"},{\"content\":{\"connectorIds\":[\"Out1\"],\"side\":\"RIGHT\"},\"type\":\"ConnectorPlacement.EquallySpacedRectSide\",\"uuid\":\"e118f150-fee7-4aeb-941e-53c3f02c6791\"},{\"content\":{\"connectorIds\":[\"Out2\"],\"side\":\"TOP\"},\"type\":\"ConnectorPlacement.EquallySpacedRectSide\",\"uuid\":\"6d9038ab-faad-455b-a9c5-8fe0bbf34e51\"},{\"content\":{\"connectorIds\":[\"In2\"],\"side\":\"BOTTOM\"},\"type\":\"ConnectorPlacement.EquallySpacedRectSide\",\"uuid\":\"d09c8d4f-08f3-4c52-88a6-8c6db517fc7a\"}]},\"type\":\"ConnectorPlacement.EquallySpacedConnector\",\"uuid\":\"5bc947ce-f1cd-4957-9186-40c14c78de7d\"}],\"packageUris\":[\"http://schema.mathworks.com/mf0/Connector/R2020b\"],\"version\":\"1.0\"}"
  Half Adder1 : Subsystem
      settings: PortSchema="{\"entries\":[{\"content\":{\"sides\":[{\"content\":{\"connectorIds\":[\"In1\"]},\"type\":\"ConnectorPlacement.EquallySpacedRectSide\",\"uuid\":\"d3a7e232-15f2-47a9-a065-9480c81dc57e\"},{\"content\":{\"connectorIds\":[\"Out1\"],\"side\":\"RIGHT\"},\"type\":\"ConnectorPlacement.EquallySpacedRectSide\",\"uuid\":\"e118f150-fee7-4aeb-941e-53c3f02c6791\"},{\"content\":{\"connectorIds\":[\"Out2\"],\"side\":\"TOP\"},\"type\":\"ConnectorPlacement.EquallySpacedRectSide\",\"uuid\":\"6d9038ab-faad-455b-a9c5-8fe0bbf34e51\"},{\"content\":{\"connectorIds\":[\"In2\"],\"side\":\"BOTTOM\"},\"type\":\"ConnectorPlacement.EquallySpacedRectSide\",\"uuid\":\"d09c8d4f-08f3-4c52-88a6-8c6db517fc7a\"}]},\"type\":\"ConnectorPlacement.EquallySpacedConnector\",\"uuid\":\"5bc947ce-f1cd-4957-9186-40c14c78de7d\"}],\"packageUris\":[\"http://schema.mathworks.com/mf0/Connector/R2020b\"],\"version\":\"1.0\"}"
  Half Adder2 : Subsystem
      settings: PortSchema="{\"entries\":[{\"content\":{\"sides\":[{\"content\":{\"connectorIds\":[\"In1\"]},\"type\":\"ConnectorPlacement.EquallySpacedRectSide\",\"uuid\":\"d3a7e232-15f2-47a9-a065-9480c81dc57e\"},{\"content\":{\"connectorIds\":[\"Out1\"],\"side\":\"RIGHT\"},\"type\":\"ConnectorPlacement.EquallySpacedRectSide\",\"uuid\":\"e118f150-fee7-4aeb-941e-53c3f02c6791\"},{\"content\":{\"connectorIds\":[\"Out2\"],\"side\":\"TOP\"},\"type\":\"ConnectorPlacement.EquallySpacedRectSide\",\"uuid\":\"6d9038ab-faad-455b-a9c5-8fe0bbf34e51\"},{\"content\":{\"connectorIds\":[\"In2\"],\"side\":\"BOTTOM\"},\"type\":\"ConnectorPlacement.EquallySpacedRectSide\",\"uuid\":\"d09c8d4f-08f3-4c52-88a6-8c6db517fc7a\"}]},\"type\":\"ConnectorPlacement.EquallySpacedConnector\",\"uuid\":\"5bc947ce-f1cd-4957-9186-40c14c78de7d\"}],\"packageUris\":[\"http://schema.mathworks.com/mf0/Connector/R2020b\"],\"version\":\"1.0\"}"
  Half Adder3 : Subsystem
      settings: PortSchema="{\"entries\":[{\"content\":{\"sides\":[{\"content\":{\"connectorIds\":[\"In1\"]},\"type\":\"ConnectorPlacement.EquallySpacedRectSide\",\"uuid\":\"d3a7e232-15f2-47a9-a065-9480c81dc57e\"},{\"content\":{\"connectorIds\":[\"Out1\"],\"side\":\"RIGHT\"},\"type\":\"ConnectorPlacement.EquallySpacedRectSide\",\"uuid\":\"e118f150-fee7-4aeb-941e-53c3f02c6791\"},{\"content\":{\"connectorIds\":[\"Out2\"],\"side\":\"TOP\"},\"type\":\"ConnectorPlacement.EquallySpacedRectSide\",\"uuid\":\"6d9038ab-faad-455b-a9c5-8fe0bbf34e51\"},{\"content\":{\"connectorIds\":[\"In2\"],\"side\":\"BOTTOM\"},\"type\":\"ConnectorPlacement.EquallySpacedRectSide\",\"uuid\":\"d09c8d4f-08f3-4c52-88a6-8c6db517fc7a\"}]},\"type\":\"ConnectorPlacement.EquallySpacedConnector\",\"uuid\":\"5bc947ce-f1cd-4957-9186-40c14c78de7d\"}],\"packageUris\":[\"http://schema.mathworks.com/mf0/Connector/R2020b\"],\"version\":\"1.0\"}"
  Half Adder4 : Subsystem
      settings: PortSchema="{\"entries\":[{\"content\":{\"sides\":[{\"content\":{\"connectorIds\":[\"In1\"]},\"type\":\"ConnectorPlacement.EquallySpacedRectSide\",\"uuid\":\"d3a7e232-15f2-47a9-a065-9480c81dc57e\"},{\"content\":{\"connectorIds\":[\"Out1\"],\"side\":\"RIGHT\"},\"type\":\"ConnectorPlacement.EquallySpacedRectSide\",\"uuid\":\"e118f150-fee7-4aeb-941e-53c3f02c6791\"},{\"content\":{\"connectorIds\":[\"Out2\"],\"side\":\"TOP\"},\"type\":\"ConnectorPlacement.EquallySpacedRectSide\",\"uuid\":\"6d9038ab-faad-455b-a9c5-8fe0bbf34e51\"},{\"content\":{\"connectorIds\":[\"In2\"],\"side\":\"BOTTOM\"},\"type\":\"ConnectorPlacement.EquallySpacedRectSide\",\"uuid\":\"d09c8d4f-08f3-4c52-88a6-8c6db517fc7a\"}]},\"type\":\"ConnectorPlacement.EquallySpacedConnector\",\"uuid\":\"5bc947ce-f1cd-4957-9186-40c14c78de7d\"}],\"packageUris\":[\"http://schema.mathworks.com/mf0/Connector/R2020b\"],\"version\":\"1.0\"}"
  Half Adder5 : Subsystem
      settings: PortSchema="{\"entries\":[{\"content\":{\"sides\":[{\"content\":{\"connectorIds\":[\"In1\"]},\"type\":\"ConnectorPlacement.EquallySpacedRectSide\",\"uuid\":\"d3a7e232-15f2-47a9-a065-9480c81dc57e\"},{\"content\":{\"connectorIds\":[\"Out1\"],\"side\":\"RIGHT\"},\"type\":\"ConnectorPlacement.EquallySpacedRectSide\",\"uuid\":\"e118f150-fee7-4aeb-941e-53c3f02c6791\"},{\"content\":{\"connectorIds\":[\"Out2\"],\"side\":\"TOP\"},\"type\":\"ConnectorPlacement.EquallySpacedRectSide\",\"uuid\":\"6d9038ab-faad-455b-a9c5-8fe0bbf34e51\"},{\"content\":{\"connectorIds\":[\"In2\"],\"side\":\"BOTTOM\"},\"type\":\"ConnectorPlacement.EquallySpacedRectSide\",\"uuid\":\"d09c8d4f-08f3-4c52-88a6-8c6db517fc7a\"}]},\"type\":\"ConnectorPlacement.EquallySpacedConnector\",\"uuid\":\"5bc947ce-f1cd-4957-9186-40c14c78de7d\"}],\"packageUris\":[\"http://schema.mathworks.com/mf0/Connector/R2020b\"],\"version\":\"1.0\"}"
  Half Adder6 : Subsystem
      settings: PortSchema="{\"entries\":[{\"content\":{\"sides\":[{\"content\":{\"connectorIds\":[\"In1\"]},\"type\":\"ConnectorPlacement.EquallySpacedRectSide\",\"uuid\":\"d3a7e232-15f2-47a9-a065-9480c81dc57e\"},{\"content\":{\"connectorIds\":[\"Out1\"],\"side\":\"RIGHT\"},\"type\":\"ConnectorPlacement.EquallySpacedRectSide\",\"uuid\":\"e118f150-fee7-4aeb-941e-53c3f02c6791\"},{\"content\":{\"side\":\"TOP\"},\"type\":\"ConnectorPlacement.EquallySpacedRectSide\",\"uuid\":\"6d9038ab-faad-455b-a9c5-8fe0bbf34e51\"},{\"content\":{\"connectorIds\":[\"In2\"],\"side\":\"BOTTOM\"},\"type\":\"ConnectorPlacement.EquallySpacedRectSide\",\"uuid\":\"d09c8d4f-08f3-4c52-88a6-8c6db517fc7a\"}]},\"type\":\"ConnectorPlacement.EquallySpacedConnector\",\"uuid\":\"5bc947ce-f1cd-4957-9186-40c14c78de7d\"}],\"packageUris\":[\"http://schema.mathworks.com/mf0/Connector/R2020b\"],\"version\":\"1.0\"}"
  Half Adder7 : Subsystem
      settings: PortSchema="{\"entries\":[{\"content\":{\"sides\":[{\"content\":{\"connectorIds\":[\"In1\"]},\"type\":\"ConnectorPlacement.EquallySpacedRectSide\",\"uuid\":\"d3a7e232-15f2-47a9-a065-9480c81dc57e\"},{\"content\":{\"connectorIds\":[\"Out1\"],\"side\":\"RIGHT\"},\"type\":\"ConnectorPlacement.EquallySpacedRectSide\",\"uuid\":\"e118f150-fee7-4aeb-941e-53c3f02c6791\"},{\"content\":{\"connectorIds\":[\"Out2\"],\"side\":\"TOP\"},\"type\":\"ConnectorPlacement.EquallySpacedRectSide\",\"uuid\":\"6d9038ab-faad-455b-a9c5-8fe0bbf34e51\"},{\"content\":{\"connectorIds\":[\"In2\"],\"side\":\"BOTTOM\"},\"type\":\"ConnectorPlacement.EquallySpacedRectSide\",\"uuid\":\"d09c8d4f-08f3-4c52-88a6-8c6db517fc7a\"}]},\"type\":\"ConnectorPlacement.EquallySpacedConnector\",\"uuid\":\"5bc947ce-f1cd-4957-9186-40c14c78de7d\"}],\"packageUris\":[\"http://schema.mathworks.com/mf0/Connector/R2020b\"],\"version\":\"1.0\"}"
  Mux1 : Mux  Inputs=8
  Mux2 : Mux  Inputs=8
  NOT : Logic  Operator=NOT  IconShape=distinctive  AllPortsSameDT=off  OutDataTypeStr=boolean
  TC : Outport
  wires:
  Mux1/1 -> Delay One Step/1
  TC_RST/1 -> NOT/1
  Delay One Step/1 -> Demux/1
  Demux/4 -> D Flip-Flop4/1
  Demux/3 -> D Flip-Flop2/1
  Demux/2 -> D Flip-Flop3/1
  Demux/1 -> D Flip-Flop1/1
  Demux/8 -> D Flip-Flop7/1
  Demux/7 -> D Flip-Flop5/1
  Demux/6 -> D Flip-Flop6/1
  Demux/5 -> D Flip-Flop11/1
  INC/1 -> D Flip-Flop2/2, D Flip-Flop3/2, D Flip-Flop1/2, D Flip-Flop4/2, D Flip-Flop11/2, D Flip-Flop6/2, D Flip-Flop5/2, D Flip-Flop7/2
  Constant/1 -> Half Adder7/2("B ")
  Half Adder5/2(Carry) -> Half Adder6/2("B ")
  Half Adder/2(Carry) -> Half Adder1/2("B ")
  Half Adder4/1(Sum) -> Mux1/3
  Half Adder6/1(Sum) -> Mux1/1
  Half Adder5/1(Sum) -> Mux1/2
  Half Adder1/1(Sum) -> Mux1/6
  Half Adder/1(Sum) -> Mux1/7
  Half Adder2/1(Sum) -> Mux1/5
  Half Adder2/2(Carry) -> Half Adder3/2("B ")
  Half Adder3/1(Sum) -> Mux1/4
  Half Adder4/2(Carry) -> Half Adder5/2("B ")
  Half Adder3/2(Carry) -> Half Adder4/2("B ")
  Half Adder1/2(Carry) -> Half Adder2/2("B ")
  Half Adder7/1(Sum) -> Mux1/8
  Half Adder7/2(Carry) -> Half Adder/2("B ")
  D Flip-Flop1/1 -> Mux2/1, Half Adder6/1(A)  "D1"
  D Flip-Flop3/1 -> Mux2/2, Half Adder5/1(A)  "D3"
  D Flip-Flop2/1 -> Mux2/3, Half Adder4/1(A)  "D4"
  D Flip-Flop4/1 -> Mux2/4, Half Adder3/1(A)  "D2"
  D Flip-Flop11/1 -> Mux2/5, Half Adder2/1(A)  "D1"
  D Flip-Flop6/1 -> Mux2/6, Half Adder1/1(A)  "D3"
  D Flip-Flop5/1 -> Mux2/7, Half Adder/1(A)  "D4"
  D Flip-Flop7/1 -> Mux2/8, Half Adder7/1(A)  "D2"
  Mux2/1 -> TC/1
  NOT/1 -> D Flip-Flop2/3, D Flip-Flop1/3, D Flip-Flop3/3, D Flip-Flop4/3, D Flip-Flop11/3, D Flip-Flop6/3, D Flip-Flop5/3, D Flip-Flop7/3
